simulink model "QuadSurge"  (R2015b)
settings: Solver=ode45  StartTime=tstart  StopTime=tstop  RelTol=1e-3
values from neighbouring files (symbols this model uses):
  n_c = elm    [AnalyseSurgeSpeed.m]    (also in SurgeDynamicsTest.m = nc_list(i); SurgeSpeedTest.m = nc_list(i); analyse_dynamics.m = nc_list(i); matlab.mat = 8.9)
  tsamp = 10    [AnalyseSpeedCharacteristis.m]    (also in AnalyseSpeedModel.m; AnalyseSurgeSpeed.m; Analyse_steadystate.m; SurgeDynamicsTest.m)
  x = lsqcurvefit(F2, x0, t, v(:,1),[],[],OPT)    [SurgeDynamicsTest.m]    (also in analyse_dynamics.m = lsqcurvefit(F3, x0, t, v(:,1),[0.09 0.2 600],[0.13 0.6 1150]; analyse_sway_dynamics.m = lsqcurvefit(F2, x0, t, v,[0 0],[],OPT))
settings Model: ExtModeAutoUpdateStatusClock=off  Creator=christh  LastModifiedBy=Erik
settings DataIOCC: SaveFormat=Array  SignalLoggingSaveFormat=ModelDataLogs
settings OptimizationCC: ExpressionDepthLimit=2147483647  InitFltsAndDblsToZero=on
settings DebuggingCC: UnderspecifiedInitializationDetection=Classic  MergeDetectMultiDrivingBlocksExec=none  SolverPrmCheckMsg=warning  FcnCallInpInsideContextMsg=UseLocalSettings  StateNameClashWarn=warning
settings HardwareCC: ProdBitPerPointer=32  ProdLargestAtomicFloat=None  ProdIntDivRoundTo=Undefined  ProdEndianess=Unspecified  ProdWordSize=32  ProdHWDeviceType=32-bit Generic
settings GRTTargetCC: GeneratePreprocessorConditionals=Disable all  CombineOutputUpdateFcns=off  GRTInterface=on
settings ConfigComp: CovModelRefEnable=Off

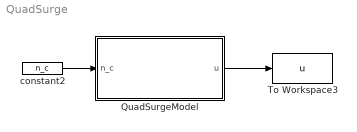
== system QuadSurge ==
  QuadSurgeModel : Subsystem
  To Workspace3 : ToWorkspace  VariableName=u  SampleTime=tsamp
  constant2 : Constant  Value=n_c
  wires:
  constant2/1 -> QuadSurgeModel/1(n_c)
  QuadSurgeModel/1(u) -> To Workspace3/1

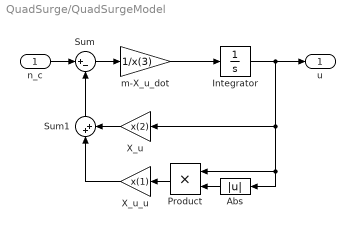
== system QuadSurge/QuadSurgeModel ==
  n_c : Inport
  Abs : Abs
  Integrator : Integrator
  Product : Product
  Sum : Sum  Inputs=|+-
  Sum1 : Sum  Inputs=|++
  X_u : Gain  Gain=x(2)
  X_u_u : Gain  Gain=x(1)
  m-X_u_dot : Gain  Gain=1/x(3)
  u : Outport
  wires:
  Sum1/1 -> Sum/2
  X_u_u/1 -> Sum1/1
  Integrator/1 -> u/1, X_u/1, Abs/1, Product/1
  n_c/1 -> Sum/1
  Abs/1 -> Product/2
  Product/1 -> X_u_u/1
  X_u/1 -> Sum1/2
  Sum/1 -> m-X_u_dot/1
  m-X_u_dot/1 -> Integrator/1
